simulink library "INT_RmtAPP_Kickdown"  (R2016b)
settings: Solver=VariableStepAuto  StartTime=0.0  StopTime=10.0  RelTol=1e-3
settings Model: Creator=xuxingpei  LastModifiedBy=xuxingpei

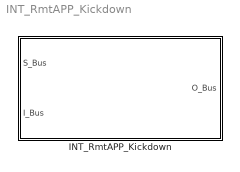
== system INT_RmtAPP_Kickdown ==
  INT_RmtAPP_Kickdown : Subsystem

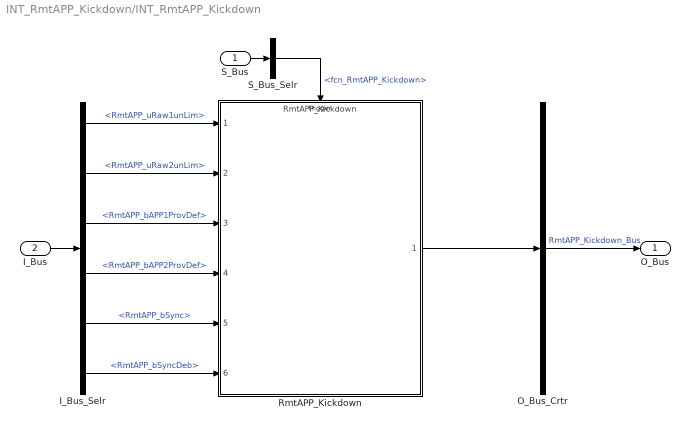
== system INT_RmtAPP_Kickdown/INT_RmtAPP_Kickdown ==
  S_Bus : Inport
  I_Bus : Inport  Port=2
  I_Bus_Selr : BusSelector  OutputSignals=RmtAPP_uRaw1unLim,RmtAPP_uRaw2unLim,RmtAPP_bAPP1ProvDef,RmtAPP_bAPP2ProvDef,RmtAPP_bSync,RmtAPP_bSyncDeb
  O_Bus_Crtr : BusCreator  Inputs=1
  RmtAPP_Kickdown : ModelReference  ModelNameDialog=RmtAPP_Kickdown  SimulationMode=Normal  ModelReferenceVersion=1.6  TriggerPortName=function  TriggerPortTriggerType=function-call  TriggerPortStatesWhenEnabling=held
  S_Bus_Selr : BusSelector  OutputSignals=fcn_RmtAPP_Kickdown
  O_Bus : Outport
  wires:
  S_Bus_Selr/1 -> RmtAPP_Kickdown/Trigger  "<fcn_RmtAPP_Kickdown>"
  S_Bus/1 -> S_Bus_Selr/1
  I_Bus/1 -> I_Bus_Selr/1
  I_Bus_Selr/1 -> RmtAPP_Kickdown/1  "<RmtAPP_uRaw1unLim>"
  I_Bus_Selr/2 -> RmtAPP_Kickdown/2  "<RmtAPP_uRaw2unLim>"
  I_Bus_Selr/3 -> RmtAPP_Kickdown/3  "<RmtAPP_bAPP1ProvDef>"
  I_Bus_Selr/4 -> RmtAPP_Kickdown/4  "<RmtAPP_bAPP2ProvDef>"
  I_Bus_Selr/5 -> RmtAPP_Kickdown/5  "<RmtAPP_bSync>"
  I_Bus_Selr/6 -> RmtAPP_Kickdown/6  "<RmtAPP_bSyncDeb>"
  O_Bus_Crtr/1 -> O_Bus/1  "RmtAPP_Kickdown_Bus"
  RmtAPP_Kickdown/1 -> O_Bus_Crtr/1
